simulink library "eci_2_ecef_lib"  (R2016b)
settings: Solver=VariableStepAuto  StartTime=0.0  StopTime=10.0  RelTol=1e-3
settings Model: Creator=Taylor  LastModifiedBy=Taylor
settings OptimizationCC: LifeSpan=inf
settings DebuggingCC: SFExecutionAtInitializationDiag=none

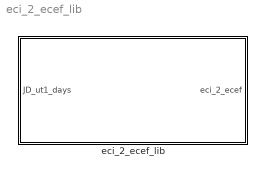
== system eci_2_ecef_lib ==
  eci_2_ecef_lib : Subsystem

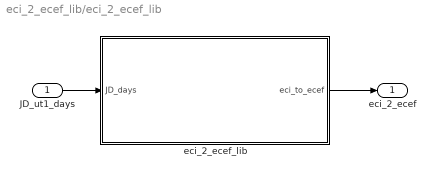
== system eci_2_ecef_lib/eci_2_ecef_lib ==
  JD_ut1_days : Inport
  eci_2_ecef_lib : MATLAB Function  TreatAsAtomicUnit=on
  eci_2_ecef : Outport
  wires:
  JD_ut1_days/1 -> eci_2_ecef_lib/1(JD_days)
  eci_2_ecef_lib/1(eci_to_ecef) -> eci_2_ecef/1

== matlab function eci_2_ecef_lib/eci_2_ecef_lib ==
  data: eci_to_ecef output; JD_days input
function eci_to_ecef = eci_to_ecef(JD_days)

% Simplified Earth rotation model

omega_e =           0.000072921158553; %[rad/s] rotation rate of Earth
theta_GMST_2000 =   1.74476716333061; % [rad]
theta_GMST =        theta_GMST_2000+omega_e*86400*(JD_days + 0.5); % [rad]

ecef_to_eci = [     cos(theta_GMST),    -sin(theta_GMST),   0;
                    sin(theta_GMST),    cos(theta_GMST),    0;
                    0,                  0,                  1];
                
eci_to_ecef =       ecef_to_eci';
